simulink model "V1VektorMatlabWs"  (R2020b)
settings: Solver=FixedStepAuto  StartTime=0.0  StopTime=20.0  FixedStep=0.1  MaxStep=0.1  MinStep=0.1  RelTol=1e-3  EnableMultiTasking=on
values from neighbouring files (symbols this model uses):
  c1 = c    (= 1)    [V1SetParam.m]    (also in V3VektorSetParam.m; V7Callback_2018_05_25_18_20_53_343.mat; V7SetParam.m; myData.mat)
  c2 = c    (= 1)    [V1SetParam.m]    (also in V3VektorSetParam.m; V7Callback_2018_05_25_18_20_53_343.mat; V7SetParam.m)
  c3 = c    (= 1)    [V1SetParam.m]    (also in V3VektorSetParam.m; V7Callback_2018_05_25_18_20_53_343.mat; V7SetParam.m)
  c4 = c    (= 1)    [V1SetParam.m]    (also in V3VektorSetParam.m; V7Callback_2018_05_25_18_20_53_343.mat; V7SetParam.m)
  m1 = m    (= 2)    [V1SetParam.m]    (also in V3VektorSetParam.m; V7Callback_2018_05_25_18_20_53_343.mat; V7SetParam.m; myData.mat)
  m2 = m    (= 2)    [V1SetParam.m]    (also in V3VektorSetParam.m; V7Callback_2018_05_25_18_20_53_343.mat; V7SetParam.m)
  m3 = m    (= 2)    [V1SetParam.m]    (also in V3VektorSetParam.m; V7Callback_2018_05_25_18_20_53_343.mat; V7SetParam.m)
  v1 = 0    [V7Callback_2018_05_25_18_20_53_343.mat]    (also in V7SetParam.m)
  v10 = 0    [V1SetParam.m]
  v20 = 0    [V1SetParam.m]
  v30 = 0    [V1SetParam.m]
  x1 = -1    [V7Callback_2018_05_25_18_20_53_343.mat]    (also in V7SetParam.m)
  x10 = -1    [V1SetParam.m]
  x20 = 0    [V1SetParam.m]
  x30 = 1    [V1SetParam.m]
settings Model: Creator=Reichl  LastModifiedBy=jakob
settings DataIOCC: SaveFormat=Array  SignalLoggingSaveFormat=ModelDataLogs  ReturnWorkspaceOutputs=off
settings OptimizationCC: ExpressionDepthLimit=2147483647  LifeSpan=inf
settings DebuggingCC: UnderspecifiedInitializationDetection=Classic  MergeDetectMultiDrivingBlocksExec=none  SolverPrmCheckMsg=warning  FcnCallInpInsideContextMsg=warning  AllowSymbolicDim=off  StateNameClashWarn=warning  SFUnexpectedBacktrackingDiag=warning  SFNoUnconditionalDefaultTransitionDiag=warning  SFExecutionAtInitializationDiag=none  ArithmeticOperatorsInVariantConditions=warning
settings HardwareCC: ProdBitPerPointer=32  ProdBitPerSizeT=32  ProdBitPerPtrDiffT=32  ProdLargestAtomicFloat=None  ProdIntDivRoundTo=Undefined  ProdEndianess=Unspecified  ProdWordSize=32  ProdHWDeviceType=32-bit Generic
settings ModelReferenceCC: PropagateSignalLabelsOutOfModel=off
settings SFSimCC: SimUseLocalCustomCode=off  CustomCodeUndefinedFunction=UseInterfaceOnly
settings RTWCC: RTWUseLocalCustomCode=off
settings CodeAppCC: StateflowObjectComments=on
settings GRTTargetCC: TargetLangStandard=C89/C90 (ANSI)  CombineOutputUpdateFcns=off  GRTInterface=on
settings ConfigComp: CovMetricSettings=dw  CovSaveCumulativeToWorkspaceVar=on  CovSaveSingleToWorkspaceVar=on  CovExternalEMLEnable=off  CovSFcnEnable=off

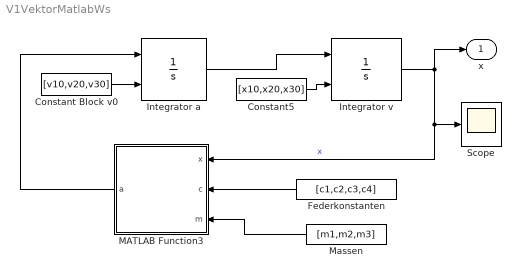
== system V1VektorMatlabWs ==
  Constant Block v0 : Constant  Value=[v10,v20,v30]
  Constant5 : Constant  Value=[x10,x20,x30]
  Federkonstanten : Constant  Value=[c1,c2,c3,c4]
  Integrator a : Integrator  InitialConditionSource=external  InitialCondition=v1
  Integrator v : Integrator  InitialConditionSource=external  InitialCondition=x1
  MATLAB Function3 : MATLAB Function  TreatAsAtomicUnit=on
  Massen : Constant  Value=[m1,m2,m3]
  Scope : Scope
  x : Outport  VectorParamsAs1DForOutWhenUnconnected=off
  wires:
  Integrator a/1 -> Integrator v/1
  Integrator v/1 -> MATLAB Function3/1(x), Scope/1, x/1  "x"
  Constant5/1 -> Integrator v/2
  Constant Block v0/1 -> Integrator a/2
  Federkonstanten/1 -> MATLAB Function3/2(c)
  Massen/1 -> MATLAB Function3/3(m)
  MATLAB Function3/1(a) -> Integrator a/1

== matlab function V1VektorMatlabWs/MATLAB Function3 ==
  data: x input size=[3,1]; a output; c input; m input
function a = fcn(x,c,m)
a=zeros(3,1); % Größe von a muss festgelegt werden
a(1,1) = -( c(1)*x(1,1) + c(2)*(x(1,1)-x(2,1)) ) / m(1);
a(2,1) = -( c(2)*(x(2,1)-x(1,1)) + c(3)*(x(2)-x(3,1)) )/m(2);
a(3,1) = -( c(3)*(x(3,1)-x(2,1)) + c(4)*x(3,1) )/m(3);
